simulink library "INT_PhyMod_PwrEntryCalc"  (R2016b)
settings: Solver=VariableStepAuto  StartTime=0.0  StopTime=10.0  RelTol=1e-3
settings Model: Creator=Administrator  LastModifiedBy=Administrator

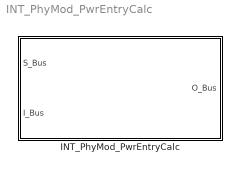
== system INT_PhyMod_PwrEntryCalc ==
  INT_PhyMod_PwrEntryCalc : Subsystem

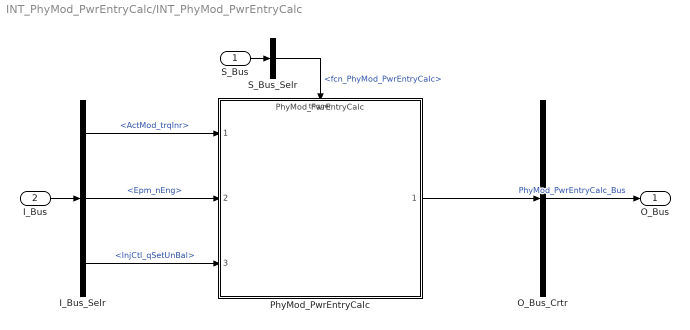
== system INT_PhyMod_PwrEntryCalc/INT_PhyMod_PwrEntryCalc ==
  S_Bus : Inport
  I_Bus : Inport  Port=2
  I_Bus_Selr : BusSelector  OutputSignals=ActMod_trqInr,Epm_nEng,InjCtl_qSetUnBal
  O_Bus_Crtr : BusCreator  Inputs=1
  PhyMod_PwrEntryCalc : ModelReference  ModelNameDialog=PhyMod_PwrEntryCalc  ModelReferenceVersion=1.1  TriggerPortName=function  TriggerPortTriggerType=function-call  TriggerPortStatesWhenEnabling=held
  S_Bus_Selr : BusSelector  OutputSignals=fcn_PhyMod_PwrEntryCalc
  O_Bus : Outport
  wires:
  S_Bus_Selr/1 -> PhyMod_PwrEntryCalc/Trigger  "<fcn_PhyMod_PwrEntryCalc>"
  S_Bus/1 -> S_Bus_Selr/1
  I_Bus/1 -> I_Bus_Selr/1
  I_Bus_Selr/1 -> PhyMod_PwrEntryCalc/1  "<ActMod_trqInr>"
  I_Bus_Selr/2 -> PhyMod_PwrEntryCalc/2  "<Epm_nEng>"
  I_Bus_Selr/3 -> PhyMod_PwrEntryCalc/3  "<InjCtl_qSetUnBal>"
  O_Bus_Crtr/1 -> O_Bus/1  "PhyMod_PwrEntryCalc_Bus"
  PhyMod_PwrEntryCalc/1 -> O_Bus_Crtr/1
